simulink model "MapBasedController"  (R2019a)
settings: Solver=VariableStepAuto  StartTime=0.0  StopTime=10.0  RelTol=1e-3
settings Model: Creator=hunter  LastModifiedBy=hunter

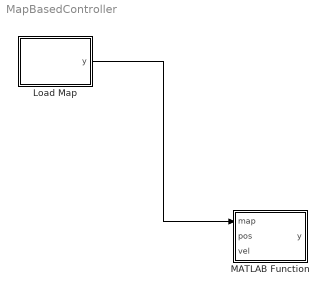
== system MapBasedController ==
  Load Map : MATLAB Function  TreatAsAtomicUnit=on
  MATLAB Function : MATLAB Function  TreatAsAtomicUnit=on
  wires:
  Load Map/1(y) -> MATLAB Function/1(map)

== matlab function MapBasedController/Load Map ==
  data: y output
function y = fcn()
    mapData = jsondecode(fileread('./markerdata/map1.json'));

    ix = mapData.inner.x.';
    iy = mapData.inner.y.';
    ox = mapData.outer.x.';
    oy = mapData.outer.y.';
    
    i = [ix; iy];
    o = [ox; oy];
    
    u = {i;o};
y = u;

== matlab function MapBasedController/MATLAB Function ==
  data: map input; pos input; y output; vel input
function y = turn(map, pos, vel)
    y = 0; %set y = 0 for no turn
    for k = 1:size(map, 1)
        for i = 2:size(map{k}, 2)
            tx = [map{k}(1, i-1) map{k}(1, i)]; %[mapData.(fields{k}).x(i-1) mapData.(fields{k}).x(i)];
            ty = [map{k}(2, i-1) map{k}(2, i)]; %[mapData.(fields{k}).y(i-1) mapData.(fields{k}).y(i)];
            plot(tx, ty, 'b-');

            q = [tx(1); ty(1)];
            s = [tx(2) - tx(1); ty(2) - ty(1)];
            
            %determine the relationship between the line segments
            t = (det(cat(2,(q - p), s)))*inv(det(cat(2, r, s)));
            u = (det(cat(2,(q - p), r)))*inv(det(cat(2, r, s)));
            
            %check for a single intersection (ignore colinear case)
            if(t >= 0 && t <= 1 && u >= 0 && u <= 1)
                %inner case, for all simple maps there will only be an
                %inner and outer case
                if(k == 1)  
                    y = 1; %turn right
                else
                    y = -1; %turn left
                end
            end
        end
    end
y = u;
